simulink model "test_pmt_input"  (Simulink 6.5)
settings: Solver=ode45  StartTime=0.0  StopTime=10.0  MaxStep=.1  RelTol=1e-3
undefined symbols (not defined in the file or in its folder): sigbuilder_block
libraries: xbsIndex_r4 x9
settings Model: Creator=nort  LastModifiedBy=nort

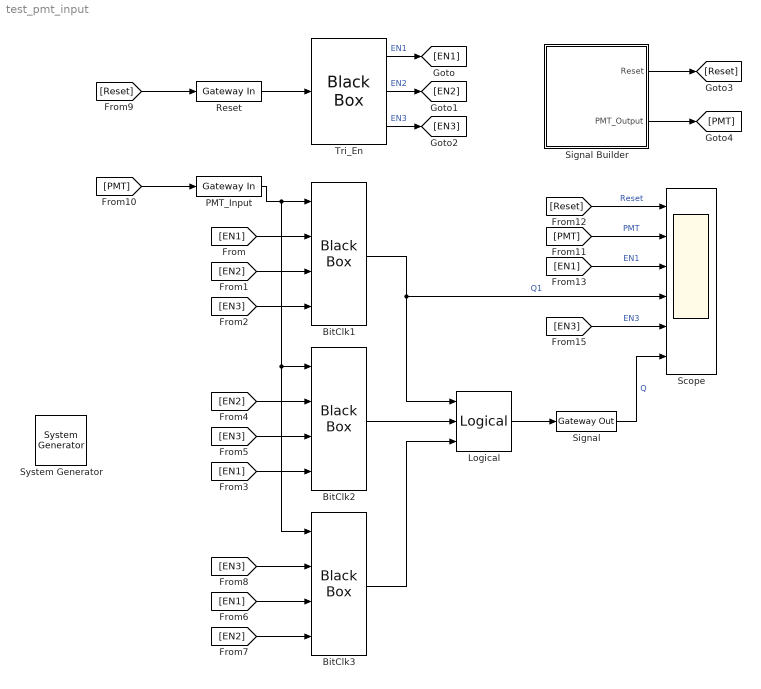
== system test_pmt_input ==
  " System Generator" : xbsIndex_r4/ System Generator  Tag=genX  SystemSampleTime=-1  xilinxfamily=virtex4  part=xc4vsx35  speed=-10  package=ff668  synthesis_tool=XST  directory=./pmt_netlist  testbench=off  simulink_period=1  sysclk_period=10  incr_netlist=off  trim_vbits=Everywhere in SubSystem  dbl_ovrd=According to Block Masks  core_generation=According to Block Masks  run_coregen=off  deprecated_control=off  eval_field=0  block_type=sysgen
      settings: block_version=9.2.01
  BitClk1 : xbsIndex_r4/Black Box  init_code=BitClk_config  sim_method=ISE Simulator  block_type=blackbox2
      settings: infoedit="Incorporates black box HDL and simulation model into a System Generator design.<P><P>You must supply a Black Box with certain information about the HDL component you would like to bring into System Generator. This information is provided through a Matlab function.<P><P>When \"Simulation mode\" is set to \"Inactive\", you will typically want to provide a separate simulation model by using a Simulation Multiplexer.<P>When \"Simulation mode\" is set to \"External co-simulator\", you must include a ModelSim block in the design."  block_version=9.2.01
  BitClk2 : xbsIndex_r4/Black Box  init_code=BitClk_config  sim_method=ISE Simulator  block_type=blackbox2
      settings: infoedit="Incorporates black box HDL and simulation model into a System Generator design.<P><P>You must supply a Black Box with certain information about the HDL component you would like to bring into System Generator. This information is provided through a Matlab function.<P><P>When \"Simulation mode\" is set to \"Inactive\", you will typically want to provide a separate simulation model by using a Simulation Multiplexer.<P>When \"Simulation mode\" is set to \"External co-simulator\", you must include a ModelSim block in the design."  block_version=9.2.01
  BitClk3 : xbsIndex_r4/Black Box  init_code=BitClk_config  sim_method=ISE Simulator  block_type=blackbox2
      settings: infoedit="Incorporates black box HDL and simulation model into a System Generator design.<P><P>You must supply a Black Box with certain information about the HDL component you would like to bring into System Generator. This information is provided through a Matlab function.<P><P>When \"Simulation mode\" is set to \"Inactive\", you will typically want to provide a separate simulation model by using a Simulation Multiplexer.<P>When \"Simulation mode\" is set to \"External co-simulator\", you must include a ModelSim block in the design."  block_version=9.2.01
  Logical : xbsIndex_r4/Logical  logical_function=OR  inputs=3  en=off  latency=0  precision=Full  arith_type=Unsigned  n_bits=16  bin_pt=0  align_bp=on  dbl_ovrd=off  block_type=logical
      settings: block_version=9.2.01
  PMT_Input : xbsIndex_r4/Gateway In  arith_type=Boolean  n_bits=1  bin_pt=0  quantization="Round  (unbiased: +/- Inf)"  overflow=Saturate  period=1  dbl_ovrd=off  timing_constraint=None  locs_specified=off  LOCs={}  block_type=gatewayin
      settings: infoedit="Gateway in block.  Converts inputs of type Simulink integer, double and fixed point to  Xilinx fixed point type.<P><P>Hardware notes:  In hardware these blocks become top level input ports."  block_version=9.2.01
  Reset : xbsIndex_r4/Gateway In  arith_type=Boolean  n_bits=1  bin_pt=0  quantization="Round  (unbiased: +/- Inf)"  overflow=Saturate  period=1  dbl_ovrd=off  timing_constraint=None  locs_specified=off  LOCs={}  block_type=gatewayin
      settings: infoedit="Gateway in block.  Converts inputs of type Simulink integer, double and fixed point to  Xilinx fixed point type.<P><P>Hardware notes:  In hardware these blocks become top level input ports."  block_version=9.2.01
  Scope : Scope  NumInputPorts=6
      settings: YMin=-5~-5~-5~-5~-5~-5  YMax=5~5~5~5~5~5
  Signal : xbsIndex_r4/Gateway Out  hdl_port=on  timing_constraint=None  locs_specified=off  LOCs={}  block_type=gatewayout
      settings: infoedit="Gateway out block.  Converts Xilinx fixed point inputs into ouputs of type Simulink integer, double, or fixed point.<P><P>Hardware notes:  In hardware these blocks become top level output ports or are discarded, depending on how they are configured."  block_version=9.2.01
  Signal Builder : Subsystem  Tag=STV Subsys  LoadFcn=sigbuilder_block('load');  StartFcn=sigbuilder_block('start');  StopFcn=sigbuilder_block('stop');  ClipboardFcn=sigbuilder_block('clipboard');  mask(Sigbuilder block){}
      mask help: Sigbuilder GUI
      mask init:
      | if ~strcmp(get_param(bdroot(gcbh),'SimulationStatus'),'stopped') tuvar = sigbuilder_block('maskInit'); end
      settings: CopyFcn=sigbuilder_block('copy');  DeleteFcn=sigbuilder_block('delete');  ModelCloseFcn=sigbuilder_block('modelClose');  PreSaveFcn=sigbuilder_block('preSave');  NameChangeFcn=sigbuilder_block('namechange');  OpenFcn=sigbuilder_block('open',[150 89.25 406.5 399.75 ]);  CloseFcn=sigbuilder_block('close');
      mask Display: plot(0,0,100,100,[10,10,40,40,10],[80,20,20,80,80],[40,10],[50,50], [40,27,10],[65,72,56],[40,25,25,10],[28,28,43,43]);
  Tri_En : xbsIndex_r4/Black Box  init_code=TRI_EN_config  sim_method=ISE Simulator  block_type=blackbox2
      settings: infoedit="Incorporates black box HDL and simulation model into a System Generator design.<P><P>You must supply a Black Box with certain information about the HDL component you would like to bring into System Generator. This information is provided through a Matlab function.<P><P>When \"Simulation mode\" is set to \"Inactive\", you will typically want to provide a separate simulation model by using a Simulation Multiplexer.<P>When \"Simulation mode\" is set to \"External co-simulator\", you must include a ModelSim block in the design."  block_version=9.2.01
  wires:
  Tri_En/1 -> [EN1]  "EN1"
  Tri_En/2 -> [EN2]  "EN2"
  Tri_En/3 -> [EN3]  "EN3"
  [EN1] -> BitClk1/2
  [EN2] -> BitClk1/3
  [EN3] -> BitClk1/4
  [EN2] -> BitClk2/2
  [EN3] -> BitClk2/3
  [EN1] -> BitClk2/4
  [EN3] -> BitClk3/2
  [EN1] -> BitClk3/3
  [EN2] -> BitClk3/4
  BitClk2/1 -> Logical/2
  BitClk1/1 -> Logical/1, Scope/4  "Q1"
  BitClk3/1 -> Logical/3
  Logical/1 -> Signal/1
  Reset/1 -> Tri_En/1
  PMT_Input/1 -> BitClk1/1, BitClk2/1, BitClk3/1
  Signal Builder/1(Reset) -> [Reset]
  Signal Builder/2(PMT_Output) -> [PMT]
  [Reset] -> Reset/1
  [PMT] -> PMT_Input/1
  [PMT] -> Scope/2  "PMT"
  [Reset] -> Scope/1  "Reset"
  [EN1] -> Scope/3  "EN1"
  [EN3] -> Scope/5  "EN3"
  Signal/1 -> Scope/6  "Q"

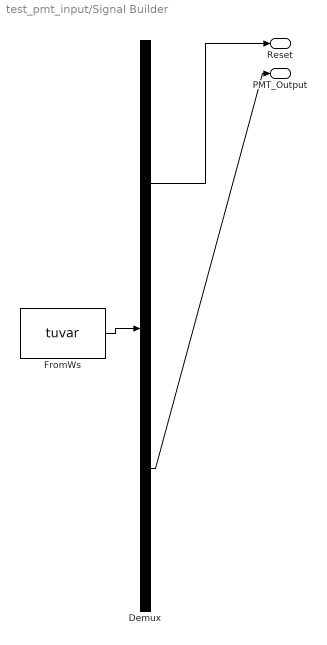
== system test_pmt_input/Signal Builder ==
  Demux : Demux  Tag=STV Demux  Outputs=2
  FromWs : FromWorkspace  Tag=STV FromWs  VariableName=tuvar  SampleTime=0  SigBuilderData=DataTag1  VnvData=DataTag2
      SigBuilderData=|
      | channels(1).label = 'Reset'
      | channels(1).allXData = {[0 1 1 10]}
      | channels(1).allYData = {[1 1 0 0]}
      | channels(2).label = 'PMT_Output'
      | channels(2).allXData = {[0 2.4 2.4 2.7 2.7 5.6 5.6 6.7 6.7 10]}
      | channels(2).allYData = {[0 0 1 1 0 0 1 1 0 0]}
      | common.afterFinalStr = 'Extrapolate'
      | common.sampleTime = 0
      | dataSet.timeRange = [0 10]
      | dataSet.name = 'Group 1'
  Reset : Outport  Tag=STV Outport
  PMT_Output : Outport  Tag=STV Outport  Port=2
  wires:
  Demux/1 -> Reset/1
  FromWs/1 -> Demux/1
  Demux/2 -> PMT_Output/1
